simulink model "Boostrapped_Switch_v2"  (R2021b)
settings: Solver=ode14x  StartTime=0.0  StopTime=103E-6  FixedStep=200E-9  RelTol=1e-3
libraries: fl_lib x8, nesl_utility x5, ee_lib x1
settings Model: Creator=mjg65  LastModifiedBy=mjg65
settings SolverCC: NumberNewtonIterations=5

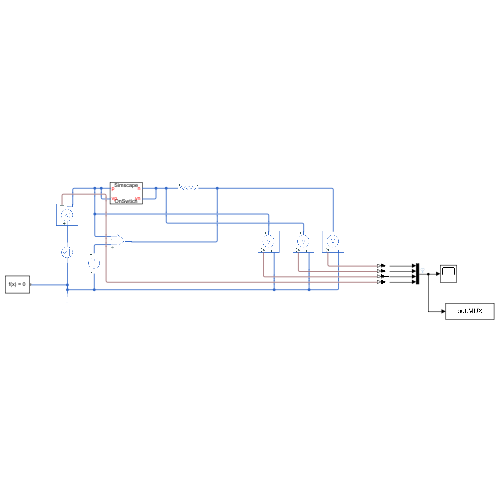
[thumbnail: Simulink's stored preview of the top-level diagram]
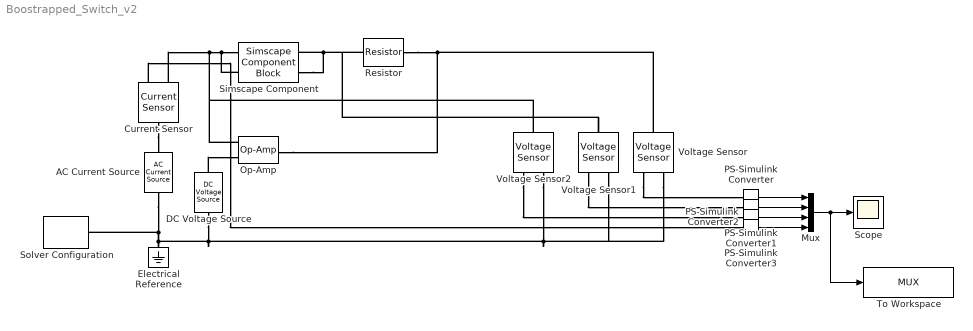
== system Boostrapped_Switch_v2 ==
  AC Current Source : fl_lib/Electrical/Electrical Sources/AC Current Source  amp=1 mA  shift=0 deg  frequency=51/512*5E6 Hz  omega=0 rad/s
      settings: SourceProductBaseCode=SS  InternalSimscapePortConfiguration="{\"Bottom\":[],\"Left\":[{\"id\":\"p\",\"label\":\"\",\"type\":\"foundation.electrical.electrical\"}],\"Right\":[{\"id\":\"n\",\"label\":\"\",\"type\":\"foundation.electrical.electrical\"}],\"Top\":[]}"
  Current Sensor : fl_lib/Electrical/Electrical Sensors/Current Sensor
  DC Voltage Source : ee_lib/Additional Components/SPICE Sources/DC Voltage Source  DC=0.9 V
  Electrical Reference : fl_lib/Electrical/Electrical Elements/Electrical Reference
  Mux : Mux
  Op-Amp : fl_lib/Electrical/Electrical Elements/Op-Amp  outI_specify=off  outI_priority=None  outI=0 A  outI_nominal_specify=off  outI_nominal_unit=A  outI_nominal_value=1
  PS-Simulink Converter{,1..3} (4 alike) : nesl_utility/PS-Simulink Converter  PhysicalDomain=network_engine_domain  SubClassName=ps_output  LeftPortType=input  RightPortType=output  PseudoPeriodic=off  Frequencies=[]  Unit=inherit  AffineConversion=off
      settings: SourceProductBaseCode=PW,SS
  Resistor : fl_lib/Electrical/Electrical Elements/Resistor  R=200 Ohm  i_specify=off  i_priority=None  i=0 A  i_nominal_specify=off  i_nominal_unit=A  i_nominal_value=1  v_specify=off  v_priority=None  v=0 V  v_nominal_specify=off  v_nominal_unit=V  v_nominal_value=1
  Scope : Scope
  Simscape Component : SimscapeComponentBlock  SourceFile=OnSwtich  ComponentPath=OnSwtich  ComponentVariants="[\"OnSwtich\"]"  ComponentVariantNames="[\"OnSwtich\"]"  ClassName=OnSwtich  SchemaVersion=1  vbs=1.8 V  vth=0.56 V  K=238.0 V^2/A  i_specify=off  i_priority=None  i=0 A  i_nominal_specify=off  i_nominal_unit=A  i_nominal_value=1  i2_specify=off  i2_priority=None  i2=0 A  i2_nominal_specify=off  i2_nominal_unit=A  i2_nominal_value=1  vsd_specify=off  vsd_priority=None  vsd=0 V  vsd_nominal_specify=off  vsd_nominal_unit=V  vsd_nominal_value=1  v_specify=off  v_priority=None  v=0 V  v_nominal_specify=off  v_nominal_unit=V  v_nominal_value=1
      settings: CopyFcn=simscape.engine.sli.internal.componentblockcallback(gcbh,'COPY')  PreCopyFcn=simscape.engine.sli.internal.componentblockcallback(gcbh,'PRECOPY')  PreDeleteFcn=simscape.engine.sli.internal.componentblockcallback(gcbh,'PREDELETE')  LogSimulationData=on  InternalSimscapePortConfiguration="{\"Bottom\":[],\"Left\":[{\"id\":\"p\",\"label\":\"p\",\"type\":\"foundation.electrical.electrical\"},{\"id\":\"vp\",\"label\":\"vp\",\"type\":\"foundation.electrical.electrical\"}],\"Right\":[{\"id\":\"n\",\"label\":\"n\",\"type\":\"foundation.electrical.electrical\"},{\"id\":\"vn\",\"label\":\"vn\",\"type\":\"foundation.electrical.electrical\"}],\"Top\":[]}"
      mask Type: OnSwtich
  Solver Configuration : nesl_utility/Solver Configuration  PhysicalDomain=network_engine_domain  SubClassName=solver  LeftPortType=input  RightPortType=generic  Tones=[]  Harmonics=[]  SimulateNoise=off  Profile=off  UseLocalSampling=off  EnableSwitchedLinearOptims=on  FrequencyDomain=off  UseCCode=off  RelTol=0.001  AbsTol=1e-06  MinStep=1e-09  ToWorkspace=off  RevertToSquareIcSolve=off  NumHomotopyIterations=100  PhasorMode=off  PhasorModeNumHarmonics=1  DoDC=off  ResidualTolerance=1e-09  UseLocalSolver=off  LocalSolverChoice=NE_BACKWARD_EULER_ADVANCER  LocalSolverSampleTime=0.001  DoFixedCost=off  MaxNonlinIter=3  MaxModeIter=2  ComputeImpulses=off  ImpulseIterations=2  LinearAlgebra=auto  EquationFormulation=NE_TIME_EF  DelaysMemoryBudget=1024  AutomaticFiltering=on  FilteringTimeConstant=0.001  PartitionStorageMethod=AS_NEEDED  PartitionMemoryBudget=1024  PartitionMethod=ROBUST
      settings: SourceProductBaseCode=PW,SS
  To Workspace : ToWorkspace  VariableName=MUX  SampleTime=-1
      settings: MaxDataPoints=512
  Voltage Sensor : fl_lib/Electrical/Electrical Sensors/Voltage Sensor
  Voltage Sensor1 : fl_lib/Electrical/Electrical Sensors/Voltage Sensor
  Voltage Sensor2 : fl_lib/Electrical/Electrical Sensors/Voltage Sensor
  wires:
  PS-Simulink Converter/1 -> Mux/1
  PS-Simulink Converter1/1 -> Mux/2
  PS-Simulink Converter2/1 -> Mux/3
  Mux/1 -> Scope/1, To Workspace/1
  PS-Simulink Converter3/1 -> Mux/4
  connections:
  Simscape Component/LConn2 -- Current Sensor/RConn2 -- Voltage Sensor2/LConn1 -- Op-Amp/LConn2 -- Simscape Component/LConn1
  AC Current Source/RConn1 -- Voltage Sensor2/RConn2 -- Voltage Sensor/RConn2 -- Voltage Sensor1/RConn2 -- DC Voltage Source/RConn1 -- Solver Configuration/RConn1 -- Electrical Reference/LConn1
  Simscape Component/RConn2 -- Voltage Sensor1/LConn1 -- Resistor/LConn1 -- Simscape Component/RConn1
  Op-Amp/RConn1 -- Voltage Sensor/LConn1 -- Resistor/RConn1
  DC Voltage Source/LConn1 -- Op-Amp/LConn1
  Voltage Sensor/RConn1 -- PS-Simulink Converter/LConn1
  Voltage Sensor1/RConn1 -- PS-Simulink Converter1/LConn1
  Voltage Sensor2/RConn1 -- PS-Simulink Converter2/LConn1
  Current Sensor/LConn1 -- AC Current Source/LConn1
  Current Sensor/RConn1 -- PS-Simulink Converter3/LConn1
